simulink model "P_3_1_f_Logisztikus_novekedes_idoeltolassal"  (R2021b)
settings: Solver=VariableStepAuto  StartTime=0.0  StopTime=35  RelTol=1e-3
settings Model: Creator=davidpaksi  LastModifiedBy=davidpaksi

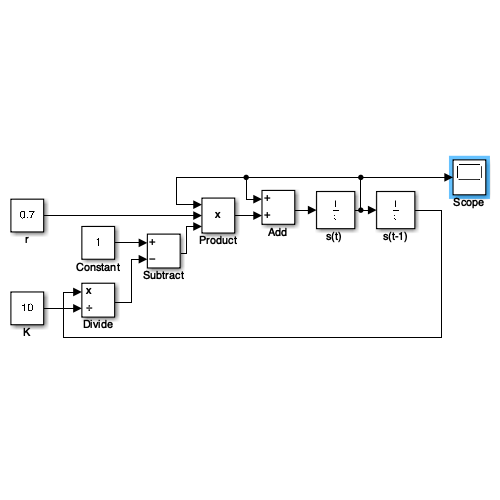
[thumbnail: Simulink's stored preview of the top-level diagram]
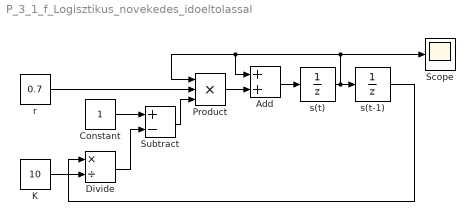
== system P_3_1_f_Logisztikus_novekedes_idoeltolassal ==
  " Add " : Sum
  " Constant " : Constant
  " Divide " : Product  Inputs=*/
  " Product " : Product  Inputs=3
  " Scope " : Scope
  " Subtract " : Sum  Inputs=+-
  K : Constant  Value=10
  r : Constant  Value=0.7
  "s(t) " : UnitDelay  InitialCondition=1  HasFrameUpgradeWarning=on
  s(t-1) : UnitDelay  HasFrameUpgradeWarning=on
  wires:
  "s(t) "/1 -> " Scope "/1, " Add "/1, " Product "/1, s(t-1)/1
  r/1 -> " Product "/2
  K/1 -> " Divide "/2
  " Constant "/1 -> " Subtract "/1
  " Divide "/1 -> " Subtract "/2
  " Subtract "/1 -> " Product "/3
  " Add "/1 -> "s(t) "/1
  " Product "/1 -> " Add "/2
  s(t-1)/1 -> " Divide "/1
